simulink library "Rectfilter_2012"  (R2016a)
settings: Solver=ode45  StartTime=0.0  StopTime=10.0  RelTol=1e-3
undefined symbols (not defined in the file): N
libraries: commfilt2 x2
settings Model: Creator=Bornitz  LastModifiedBy=Bornitz
settings DataIOCC: LimitDataPoints=on  SaveFormat=Array
settings OptimizationCC: ExpressionDepthLimit=2147483647
settings DebuggingCC: UnderspecifiedInitializationDetection=Classic  MergeDetectMultiDrivingBlocksExec=none  SolverPrmCheckMsg=warning  StateNameClashWarn=warning
settings HardwareCC: ProdBitPerPointer=32  ProdLargestAtomicFloat=None  ProdIntDivRoundTo=Undefined  ProdEndianess=Unspecified  ProdWordSize=32  ProdHWDeviceType=32-bit Generic
settings ModelReferenceCC: PropagateSignalLabelsOutOfModel=off
settings ConfigComp: CovModelRefEnable=Off

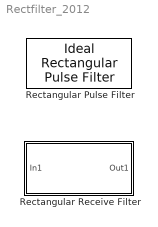
== system Rectfilter_2012 ==
  Rectangular Pulse Filter : commfilt2/Ideal Rectangular Pulse Filter  pulseLen=16  pulseDelay=0  InputProcessing=Columns as channels (frame based)  RateOptions=Allow multirate processing  sampMode=Mute  normCheck=off  normMode=Sum of samples  filterGain=1  saveAsFlag=0  roundingMode=Floor  overflowMode=off  firstCoeffDataTypeStr=Inherit: Same word length as input  firstCoeffMin=[]  firstCoeffMax=[]  firstCoeffLastDataTypeStr=Inherit: Same word length as input  outputDataTypeStr=Inherit: Same as accumulator  outputMin=[]  outputMax=[]  outputLastDataTypeStr=Inherit: Same as accumulator
  Rectangular Receive Filter : Subsystem  mask{N=N}
      mask prompts: N "Anzahl Samples/ Symbol"
      mask help:
      | Block führt eine Rechteckfilterung eines Signals durch. Die Operation
      | entspricht einem Running Mean über N Abtastwerte.
      mask Help:
      | Block führt eine Rechteckfilterung eines Signals durch. Die Operation
      | entspricht einem Running Mean über N Abtastwerte.
      | 
      | !!Definition der Länge N des Symbols notwendig!!
      mask Display:
      | plot(0,0,100,100,[95 5 10 10 10 reshape(([85*[0:1/15:1-1/15]+10; 85*[1/15:1/15:1]+10]),1,30)],[75 75 75 70 95 90 90 90 90 90 90 90 90 80 80 80 80 80 80 80 80 80 80 90 90 90 90 90 90 90 90 80 80 80 80]*1.1-10);
      | text(50,35,'Rectangular\nReceive Filter','horiz','center');

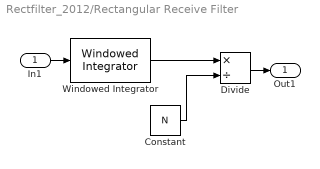
== system Rectfilter_2012/Rectangular Receive Filter ==
  In1 : Inport
  Constant : Constant  Value=N
  Divide : Product  Inputs=*/
  Windowed Integrator : commfilt2/Windowed Integrator  integperiod=N  roundingMode=Floor  overflowMode=off  InputProcessing=Columns as channels (frame based)
  Out1 : Outport
  wires:
  Constant/1 -> Divide/2
  In1/1 -> Windowed Integrator/1
  Divide/1 -> Out1/1
  Windowed Integrator/1 -> Divide/1
